simulink model "BLDC"  (R2022b)
settings: Solver=FixedStepAuto  StartTime=0.0  StopTime=10.0  RelTol=1e-3
settings Model: Creator=yuzehong  LastModifiedBy=程一帆
settings OptimizationCC: DefaultParameterBehavior=Inlined  UseDivisionForNetSlopeComputation=on  GainParamInheritBuiltInType=on  UseFloatMulNetSlope=on  InlineInvariantSignals=on  ReuseModelBlockBuffer=on  PassReuseOutputArgsAs=Individual arguments  NoFixptDivByZeroProtection=on  EfficientFloat2IntCast=on  LifeSpan=1  OptimizeBlockOrder=speed  DifferentSizesBufferReuse=on  EfficientTunableParamExpr=on
settings DebuggingCC: ParameterTunabilityLossMsg=error
settings HardwareCC: ProdLongLongMode=on
settings SFSimCC: MATLABDynamicMemAlloc=off
settings RTWCC: Description=Embedded Coder  SystemTargetFile=ert.tlc  GenCodeOnly=on  TemplateMakefile=ert_default_tmf  GPUComputeCapability=5.0
settings CodeAppCC: GenerateComments=off  IgnoreCustomStorageClasses=off  OperatorAnnotations=on  SimulinkDataObjDesc=on  SFDataObjDesc=on  CustomSymbolStrGlobalVar=rt$N$M  CustomSymbolStrType=$N$M  CustomSymbolStrFcn=$N$M$F  CustomSymbolStrMacro=$N$M  SimulinkBlockComments=off
settings ERTTargetCC: TargetLangStandard=C99 (ISO)  GenerateSampleERTMain=on  IncludeMdlTerminateFcn=off  CombineSignalStateStructs=on  SupportAbsoluteTime=off  CodeInterfacePackaging=Reusable function  SupportComplex=off  SupportContinuousTime=on  InlinedParameterPlacement=NonHierarchical  ERTCustomFileTemplate=example_file_process.tlc  ERTFilePackagingFormat=CompactWithDataFile

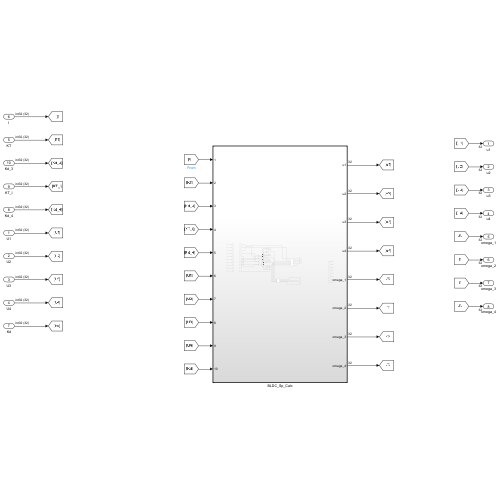
[thumbnail: Simulink's stored preview of the top-level diagram]
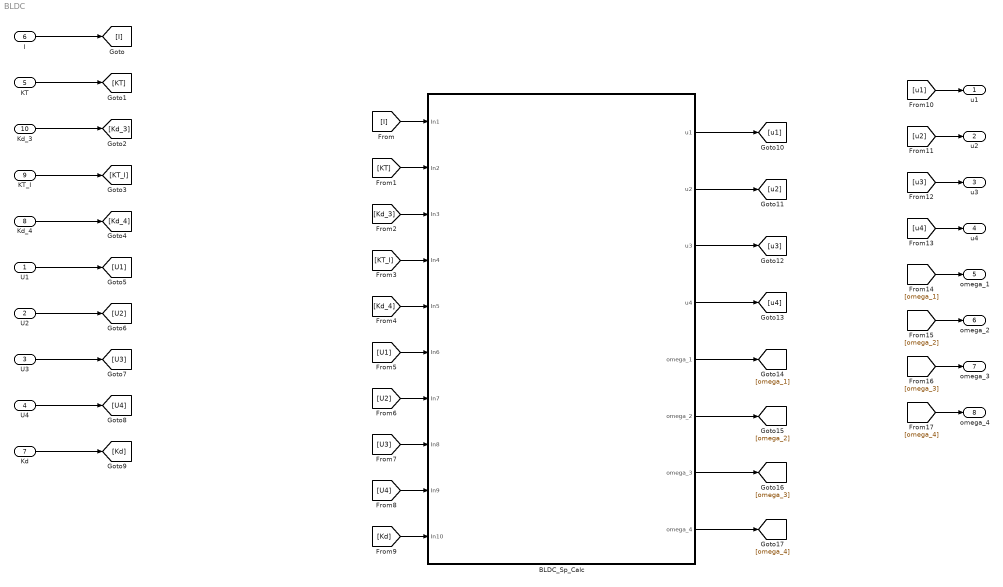
== system BLDC ==
  U1 : Inport  OutDataTypeStr=int32  PortDimensions=32
  U2 : Inport  Port=2  OutDataTypeStr=int32  PortDimensions=32
  U3 : Inport  Port=3  OutDataTypeStr=int32  PortDimensions=32
  U4 : Inport  Port=4  OutDataTypeStr=int32  PortDimensions=32
  KT : Inport  Port=5  OutDataTypeStr=int32  PortDimensions=32
  I : Inport  Port=6  OutDataTypeStr=int32  PortDimensions=32
  Kd : Inport  Port=7  OutDataTypeStr=int32  PortDimensions=32
  Kd_4 : Inport  Port=8  OutDataTypeStr=int32  PortDimensions=32
  KT_I : Inport  Port=9  OutDataTypeStr=int32  PortDimensions=32
  Kd_3 : Inport  Port=10  OutDataTypeStr=int32  PortDimensions=32
  BLDC_Sp_Calc : Subsystem  TreatAsAtomicUnit=on
      settings: RTWFcnNameOpts=Use subsystem name
  u1 : Outport  PortDimensions=32  VectorParamsAs1DForOutWhenUnconnected=off
  u2 : Outport  Port=2  PortDimensions=32  VectorParamsAs1DForOutWhenUnconnected=off
  u3 : Outport  Port=3  PortDimensions=32  VectorParamsAs1DForOutWhenUnconnected=off
  u4 : Outport  Port=4  PortDimensions=32  VectorParamsAs1DForOutWhenUnconnected=off
  omega_1 : Outport  Port=5  PortDimensions=32  VectorParamsAs1DForOutWhenUnconnected=off
  omega_2 : Outport  Port=6  PortDimensions=32  VectorParamsAs1DForOutWhenUnconnected=off
  omega_3 : Outport  Port=7  PortDimensions=32  VectorParamsAs1DForOutWhenUnconnected=off
  omega_4 : Outport  Port=8  PortDimensions=32  VectorParamsAs1DForOutWhenUnconnected=off
  wires:
  I/1 -> [I]
  KT/1 -> [KT]
  Kd_3/1 -> [Kd_3]
  KT_I/1 -> [KT_I]
  Kd_4/1 -> [Kd_4]
  U1/1 -> [U1]
  U2/1 -> [U2]
  U3/1 -> [U3]
  U4/1 -> [U4]
  Kd/1 -> [Kd]
  [omega_2] -> omega_2/1
  [u1] -> u1/1
  [u4] -> u4/1
  [u3] -> u3/1
  [omega_1] -> omega_1/1
  [u2] -> u2/1
  [omega_4] -> omega_4/1
  [omega_3] -> omega_3/1
  [I] -> BLDC_Sp_Calc/1(In1)
  [KT] -> BLDC_Sp_Calc/2(In2)
  [Kd_3] -> BLDC_Sp_Calc/3(In3)
  [KT_I] -> BLDC_Sp_Calc/4(In4)
  [Kd_4] -> BLDC_Sp_Calc/5(In5)
  [U1] -> BLDC_Sp_Calc/6(In6)
  [U2] -> BLDC_Sp_Calc/7(In7)
  [U3] -> BLDC_Sp_Calc/8(In8)
  [U4] -> BLDC_Sp_Calc/9(In9)
  [Kd] -> BLDC_Sp_Calc/10(In10)
  BLDC_Sp_Calc/1(u1) -> [u1]
  BLDC_Sp_Calc/2(u2) -> [u2]
  BLDC_Sp_Calc/3(u3) -> [u3]
  BLDC_Sp_Calc/4(u4) -> [u4]
  BLDC_Sp_Calc/5(omega_1) -> [omega_1]
  BLDC_Sp_Calc/6(omega_2) -> [omega_2]
  BLDC_Sp_Calc/7(omega_3) -> [omega_3]
  BLDC_Sp_Calc/8(omega_4) -> [omega_4]

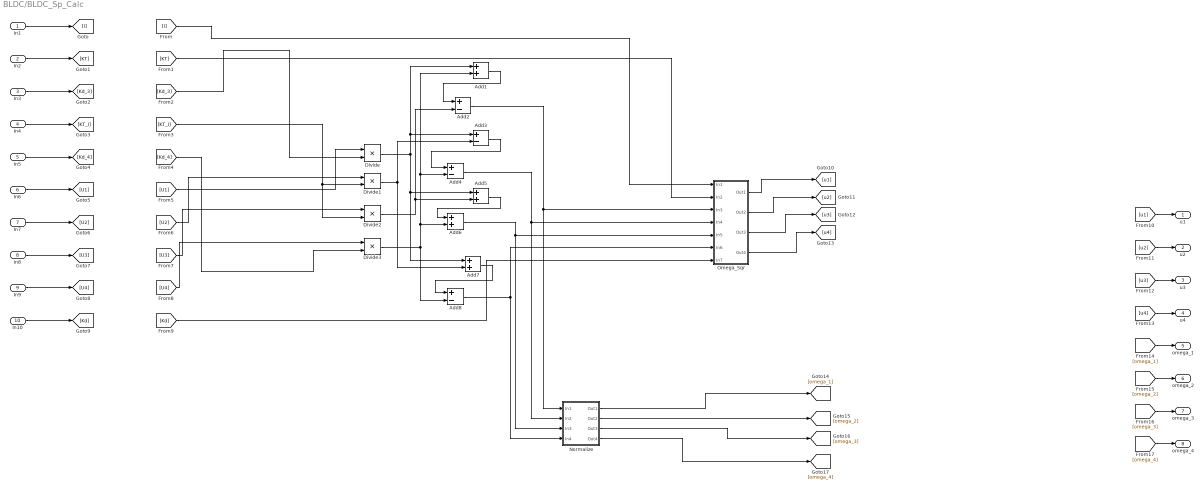
== system BLDC/BLDC_Sp_Calc ==
  In1 : Inport
  In2 : Inport  Port=2
  In3 : Inport  Port=3
  In4 : Inport  Port=4
  In5 : Inport  Port=5
  In6 : Inport  Port=6
  In7 : Inport  Port=7
  In8 : Inport  Port=8
  In9 : Inport  Port=9
  In10 : Inport  Port=10
  Add{1,5..7} (4 alike) : Sum  SaturateOnIntegerOverflow=on
  Add{2..4,8} (4 alike) : Sum  Inputs=+-  SaturateOnIntegerOverflow=on
  Divide{,1..3} (4 alike) : Product  Inputs=**  OutDataTypeStr=int32
  Normalize : Subsystem  TreatAsAtomicUnit=on
      settings: RTWFcnNameOpts=Use subsystem name
  Omega_Sqr : Subsystem  TreatAsAtomicUnit=on
      settings: RTWFcnNameOpts=Use subsystem name
  u1 : Outport  PortDimensions=32  VectorParamsAs1DForOutWhenUnconnected=off
  u2 : Outport  Port=2  PortDimensions=32  VectorParamsAs1DForOutWhenUnconnected=off
  u3 : Outport  Port=3  PortDimensions=32  VectorParamsAs1DForOutWhenUnconnected=off
  u4 : Outport  Port=4  PortDimensions=32  VectorParamsAs1DForOutWhenUnconnected=off
  omega_1 : Outport  Port=5  PortDimensions=32  VectorParamsAs1DForOutWhenUnconnected=off
  omega_2 : Outport  Port=6  PortDimensions=32  VectorParamsAs1DForOutWhenUnconnected=off
  omega_3 : Outport  Port=7  PortDimensions=32  VectorParamsAs1DForOutWhenUnconnected=off
  omega_4 : Outport  Port=8  PortDimensions=32  VectorParamsAs1DForOutWhenUnconnected=off
  wires:
  Add4/1 -> Omega_Sqr/4(In4), Normalize/2(In2)
  Divide1/1 -> Add7/2, Add3/2
  Add1/1 -> Add2/1
  Divide2/1 -> Add5/2, Add2/2
  Divide/1 -> Add3/1, Add1/1, Add7/1, Add5/1
  [U1] -> Divide/1
  Add6/1 -> Omega_Sqr/5(In5), Normalize/3(In3)
  Add8/1 -> Omega_Sqr/6(In6), Normalize/4(In4)
  [Kd_3] -> Divide/2
  Divide3/1 -> Add8/2, Add1/2, Add4/2, Add6/2
  [KT_I] -> Divide2/2, Divide1/2
  [U3] -> Divide2/1
  Add2/1 -> Omega_Sqr/3(In3), Normalize/1(In1)
  Add5/1 -> Add6/1
  Add3/1 -> Add4/1
  [U2] -> Divide1/1
  Add7/1 -> Add8/1
  [Kd_4] -> Divide3/2
  [U4] -> Divide3/1
  [I] -> Omega_Sqr/1(In1)
  [KT] -> Omega_Sqr/2(In2)
  [Kd] -> Omega_Sqr/7(In7)
  In6/1 -> [U1]
  In5/1 -> [Kd_4]
  In9/1 -> [U4]
  In4/1 -> [KT_I]
  In3/1 -> [Kd_3]
  In10/1 -> [Kd]
  In7/1 -> [U2]
  In1/1 -> [I]
  In8/1 -> [U3]
  In2/1 -> [KT]
  Normalize/1(Out1) -> [omega_1]
  Omega_Sqr/1(Out1) -> [u1]
  Omega_Sqr/3(Out3) -> [u3]
  Omega_Sqr/4(Out4) -> [u4]
  Normalize/3(Out3) -> [omega_3]
  Omega_Sqr/2(Out2) -> [u2]
  Normalize/2(Out2) -> [omega_2]
  Normalize/4(Out4) -> [omega_4]
  [omega_1] -> omega_1/1
  [u4] -> u4/1
  [omega_4] -> omega_4/1
  [u2] -> u2/1
  [omega_2] -> omega_2/1
  [u1] -> u1/1
  [u3] -> u3/1
  [omega_3] -> omega_3/1

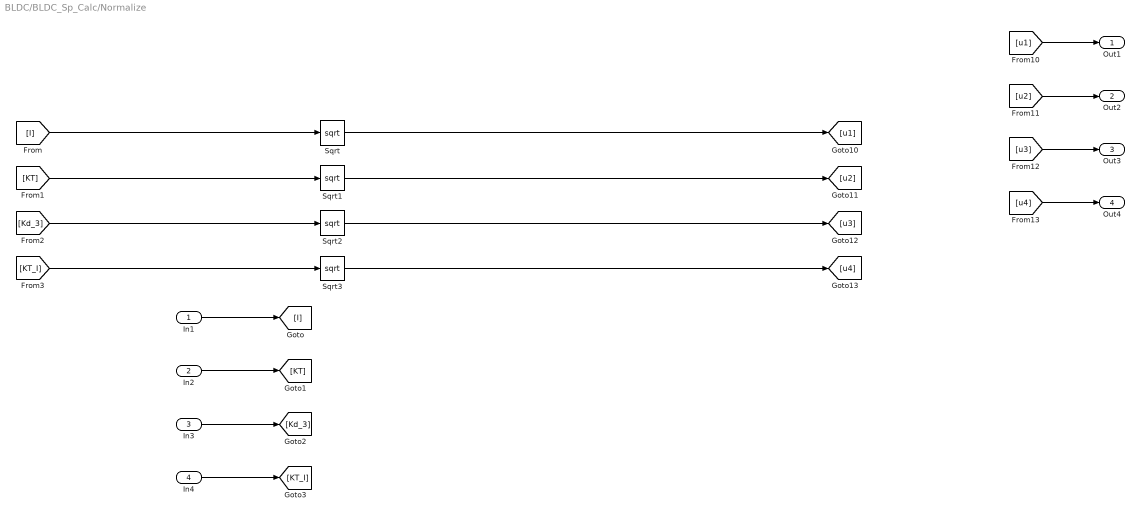
== system BLDC/BLDC_Sp_Calc/Normalize ==
  In1 : Inport
  In2 : Inport  Port=2
  In3 : Inport  Port=3
  In4 : Inport  Port=4
  Sqrt{,1..3} (4 alike) : Sqrt  OutDataTypeStr=single  SaturateOnIntegerOverflow=off
  Out1 : Outport
  Out2 : Outport  Port=2
  Out3 : Outport  Port=3
  Out4 : Outport  Port=4
  wires:
  Sqrt/1 -> [u1]
  Sqrt1/1 -> [u2]
  [KT] -> Sqrt1/1
  Sqrt2/1 -> [u3]
  [Kd_3] -> Sqrt2/1
  [KT_I] -> Sqrt3/1
  [I] -> Sqrt/1
  Sqrt3/1 -> [u4]
  In4/1 -> [KT_I]
  In3/1 -> [Kd_3]
  In1/1 -> [I]
  In2/1 -> [KT]
  [u1] -> Out1/1
  [u2] -> Out2/1
  [u3] -> Out3/1
  [u4] -> Out4/1

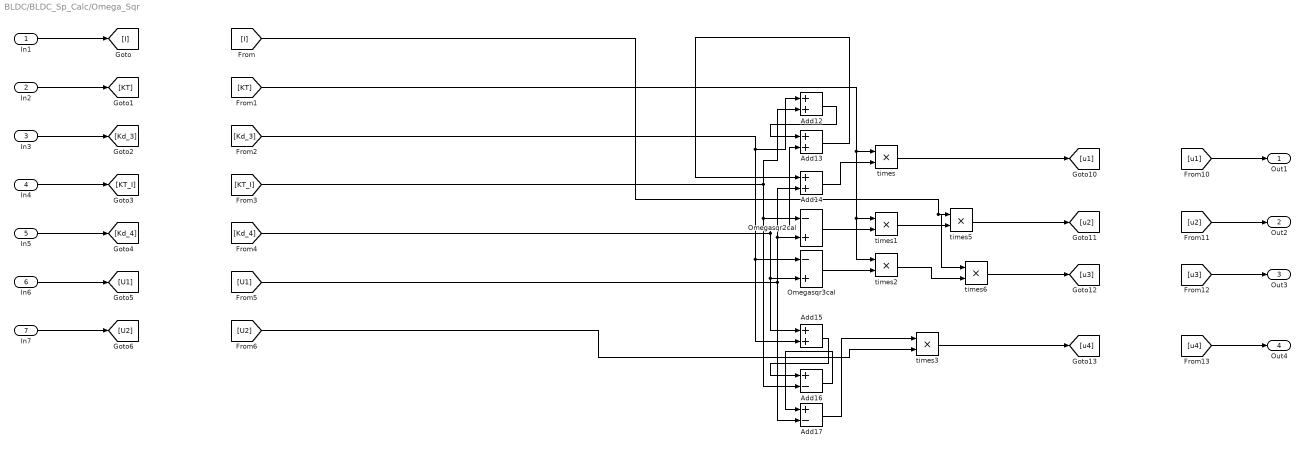
== system BLDC/BLDC_Sp_Calc/Omega_Sqr ==
  In1 : Inport
  In2 : Inport  Port=2
  In3 : Inport  Port=3
  In4 : Inport  Port=4
  In5 : Inport  Port=5
  In6 : Inport  Port=6
  In7 : Inport  Port=7
  Add{12..15} (4 alike) : Sum  SaturateOnIntegerOverflow=on
  Add16 : Sum  Inputs=+-  SaturateOnIntegerOverflow=on
  Add17 : Sum  Inputs=+-  SaturateOnIntegerOverflow=on
  Omegasqr2cal : Sum  Inputs=-+  SaturateOnIntegerOverflow=on
  Omegasqr3cal : Sum  Inputs=-+  SaturateOnIntegerOverflow=on
  times : Product  Inputs=**  OutDataTypeStr=int32
  times1 : Product  Inputs=**  OutDataTypeStr=int32
  times2 : Product  Inputs=**  OutDataTypeStr=int32
  times3 : Product  Inputs=**  OutDataTypeStr=int32  SaturateOnIntegerOverflow=on
  times5 : Product  Inputs=**  OutDataTypeStr=int32  SaturateOnIntegerOverflow=on
  times6 : Product  Inputs=**  OutDataTypeStr=int32  SaturateOnIntegerOverflow=on
  Out1 : Outport
  Out2 : Outport  Port=2
  Out3 : Outport  Port=3
  Out4 : Outport  Port=4
  wires:
  times1/1 -> times5/2
  Add15/1 -> Add16/1
  [I] -> times6/1, times5/1
  times6/1 -> [u3]
  [Kd_3] -> Add15/2, Omegasqr3cal/1, Add12/1
  Add13/1 -> Add14/1
  [U2] -> times3/2
  [KT_I] -> Omegasqr2cal/1, Add16/2, Add12/2
  [KT] -> times2/1, times1/1, times/1
  Add12/1 -> Add13/1
  [Kd_4] -> Add15/1, Omegasqr3cal/2, Add13/2
  Omegasqr3cal/1 -> times2/2
  Add14/1 -> times/2
  [U1] -> Add17/2, Add14/2, Omegasqr2cal/2
  Add17/1 -> times3/1
  times3/1 -> [u4]
  times2/1 -> times6/2
  Add16/1 -> Add17/1
  Omegasqr2cal/1 -> times1/2
  times/1 -> [u1]
  times5/1 -> [u2]
  In5/1 -> [Kd_4]
  In4/1 -> [KT_I]
  In3/1 -> [Kd_3]
  In1/1 -> [I]
  In2/1 -> [KT]
  In7/1 -> [U2]
  In6/1 -> [U1]
  [u1] -> Out1/1
  [u2] -> Out2/1
  [u3] -> Out3/1
  [u4] -> Out4/1
